simulink subsystem "Attitude_Determination"  (R2022b)
settings: Solver=VariableStepAuto  StartTime=0.0  StopTime=10.0  RelTol=1e-3
undefined symbols (not defined in the file or in its folder): catalogue, sensors, settings
libraries: simulink x1, simulink_extras x1
settings Model: Creator=Nicolò  LastModifiedBy=brent

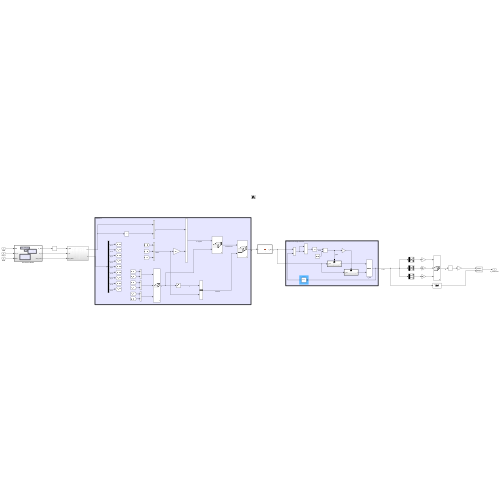
[thumbnail: Simulink's stored preview of the top-level diagram]
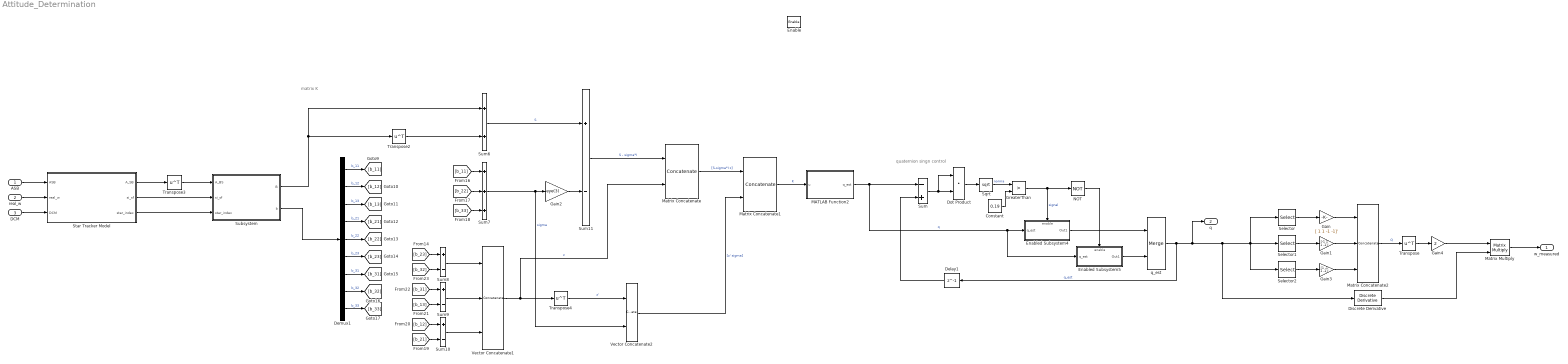
== system Attitude_Determination ==
  note: matrix K
  note: quaternion singn control
  ASB : Inport
  real_w : Inport  Port=2
  DCM : Inport  Port=3
  Enable : EnablePort
  Constant : Constant  Value=0.19
  Delay1 : Delay  DelayLength=1  InitialCondition=settings.q0
  Demux1 : Demux  Outputs=9
  Discrete Derivative : simulink/Discrete/Discrete Derivative  gainval=1.0  ICPrevScaledInput=0  OutMin=[]  OutMax=[]  OutDataType=fixdt(1, 16)  OutScaling=2^-10  DoSatur=off
  Dot Product : DotProduct  OutDataTypeStr=Inherit: Inherit via internal rule
  Enabled Subsystem4 : Subsystem  TreatAsAtomicUnit=on
  Enabled Subsystem5 : Subsystem  TreatAsAtomicUnit=on
  Gain : Gain  Gain=[ 1 1 -1 -1]'
  Gain1 : Gain  Gain=[-1 1 1 -1]'
  Gain2 : Gain  Gain=eye(3)
  Gain3 : Gain  Gain=[1 -1 1 -1]'
  Gain4 : Gain  Gain=2
  GreaterThan : RelationalOperator  Operator=>  OutDataTypeStr=boolean  RndMeth=Simplest  InputSameDT=off
  MATLAB Function2 : MATLAB Function  TreatAsAtomicUnit=on
  Matrix Concatenate : Concatenate  Mode=Multidimensional array  ConcatenateDimension=2
  Matrix Concatenate1 : Concatenate  Mode=Multidimensional array
  Matrix Concatenate2 : Concatenate  NumInputs=3  Mode=Multidimensional array  ConcatenateDimension=2
  Matrix Multiply : Product  Multiplication=Matrix(*)
  NOT : Logic  Operator=NOT  IconShape=distinctive  AllPortsSameDT=off  OutDataTypeStr=boolean
  Selector : Selector  InputPortWidth=4  IndexOptions=Index vector (dialog)  Indices=[4 3 2 1]  OutputSizes=1
  Selector1 : Selector  InputPortWidth=4  IndexOptions=Index vector (dialog)  Indices=[3 4 1 2]  OutputSizes=1
  Selector2 : Selector  InputPortWidth=4  IndexOptions=Index vector (dialog)  Indices=[2 1 4 3]  OutputSizes=1
  Sqrt : Sqrt
  Star Tracker Model : Subsystem  TreatAsAtomicUnit=on
  Subsystem : Subsystem
  Sum : Sum  Inputs=-+
  Sum{8..11} (4 alike) : Sum  Inputs=+-
  Sum6 : Sum
  Sum7 : Sum  Inputs=+++
  Transpose{,2..4} (4 alike) : Math  Operator=transpose
  Vector Concatenate1 : Concatenate  NumInputs=3  Mode=Multidimensional array
  Vector Concatenate2 : Concatenate
  q_est : Merge
  w_measured : Outport
  q : Outport  Port=2
  wires:
  Subsystem/2(b) -> Demux1/1
  Star Tracker Model/3(star_index) -> Subsystem/3(star_index)
  Constant/1 -> GreaterThan/2
  Enabled Subsystem4/1(Out1) -> q_est/1
  Demux1/2 -> [b_12]  "b_12"
  GreaterThan/1 -> NOT/1, Enabled Subsystem4/Enable  "signal"
  Gain2/1 -> Sum11/2
  Matrix Concatenate/1 -> Matrix Concatenate1/1  "[S-sigma*I z]"
  MATLAB Function2/1(q_est) -> Enabled Subsystem4/1(q_est), Enabled Subsystem5/1(q_est), Sum/1  "q"
  Sqrt/1 -> GreaterThan/1  "norma"
  Sum9/1 -> Vector Concatenate1/2
  Dot Product/1 -> Sqrt/1
  [b_32] -> Sum8/2
  Transpose4/1 -> Vector Concatenate2/1  "z'"
  NOT/1 -> Enabled Subsystem5/Enable
  Transpose2/1 -> Sum6/2
  Demux1/7 -> [b_31]  "b_31"
  Demux1/4 -> [b_21]  "b_21"
  Star Tracker Model/1(A_SB) -> Transpose3/1
  Demux1/1 -> [b_11]  "b_11"
  Sum8/1 -> Vector Concatenate1/1
  Transpose3/1 -> Subsystem/1(A_BS)
  [b_23] -> Sum8/1
  Matrix Concatenate1/1 -> MATLAB Function2/1(u)  "K"
  [b_21] -> Sum10/2
  Vector Concatenate1/1 -> Matrix Concatenate/2, Transpose4/1  "z"
  Delay1/1 -> Sum/2
  Demux1/3 -> [b_13]  "b_13"
  [b_13] -> Sum9/2
  Vector Concatenate2/1 -> Matrix Concatenate1/2  "[z' sigma]"
  [b_33] -> Sum7/3
  Sum11/1 -> Matrix Concatenate/1  "S - sigma*I"
  [b_12] -> Sum10/1
  Demux1/8 -> [b_32]  "b_32"
  Sum7/1 -> Vector Concatenate2/2, Gain2/1  "sigma"
  Demux1/9 -> [b_33]  "b_33"
  Demux1/6 -> [b_23]  "b_23"
  Demux1/5 -> [b_22]  "b_22"
  Star Tracker Model/2(si_sf) -> Subsystem/2(si_sf)
  [b_11] -> Sum7/1
  [b_22] -> Sum7/2
  Sum10/1 -> Vector Concatenate1/3
  Sum6/1 -> Sum11/1  "S"
  Subsystem/1(B) -> Sum6/1, Transpose2/1
  Sum/1 -> Dot Product/1, Dot Product/2
  Enabled Subsystem5/1(Out1) -> q_est/2
  [b_31] -> Sum9/1
  Selector2/1 -> Gain3/1
  Discrete Derivative/1 -> Matrix Multiply/2
  q_est/1 -> Discrete Derivative/1, Selector/1, Selector2/1, Selector1/1, q/1, Delay1/1  "q_est"
  Gain3/1 -> Matrix Concatenate2/3
  Matrix Concatenate2/1 -> Transpose/1  "Q"
  Selector/1 -> Gain/1
  Gain4/1 -> Matrix Multiply/1
  Matrix Multiply/1 -> w_measured/1
  Gain/1 -> Matrix Concatenate2/1
  Gain1/1 -> Matrix Concatenate2/2
  Selector1/1 -> Gain1/1
  Transpose/1 -> Gain4/1
  ASB/1 -> Star Tracker Model/1(ASB)
  real_w/1 -> Star Tracker Model/2(real_w)
  DCM/1 -> Star Tracker Model/3(DCM)

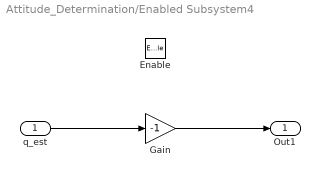
== system Attitude_Determination/Enabled Subsystem4 ==
  q_est : Inport
  Enable : EnablePort
  Gain : Gain  Gain=-1
  Out1 : Outport
  wires:
  q_est/1 -> Gain/1
  Gain/1 -> Out1/1

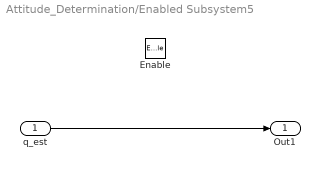
== system Attitude_Determination/Enabled Subsystem5 ==
  q_est : Inport
  Enable : EnablePort
  Out1 : Outport
  wires:
  q_est/1 -> Out1/1

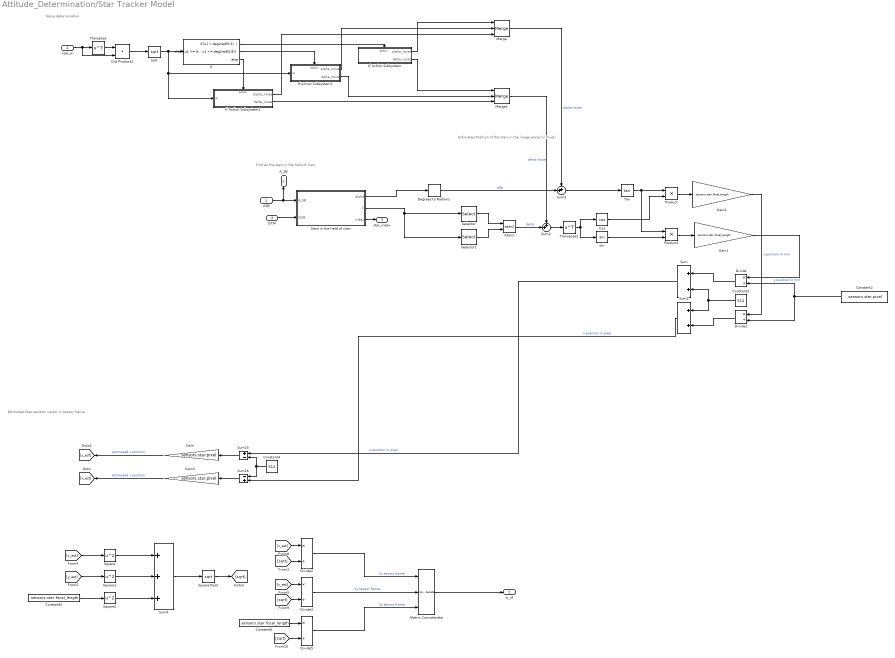
== system Attitude_Determination/Star Tracker Model ==
  note: Estimated Star position vector in Sensor frame
  note: Find all the stars in the field of view
  note: Estimated Position of the stars in the image plane (in Pixel)
  note: Noise determination
  ASB : Inport
  real_w : Inport  Port=2
  DCM : Inport  Port=3
  Atan2 : Trigonometry  Operator=atan2
  Constant2 : Constant  Value=sensors.star.pixel
  Constant3 : Constant  Value=512
  Constant4 : Constant  Value=512
  Constant5 : Constant  Value=sensors.star.focal_length
  Constant6 : Constant  Value=sensors.star.focal_length
  Cos : Trigonometry  Operator=cos
  Degrees to Radians : simulink_extras/Transformations/Degrees to Radians
  Divide{,1..3,5} (5 alike) : Product  Inputs=*/
  Dot Product2 : DotProduct  OutDataTypeStr=Inherit: Inherit via internal rule
  Gain : Gain  Gain=sensors.star.pixel
  Gain1 : Gain  Gain=sensors.star.focal_length
  Gain2 : Gain  Gain=sensors.star.focal_length
  Gain3 : Gain  Gain=sensors.star.pixel
  If : If  IfExpression=u1 < deg2rad(0.3)  ElseIfExpressions="u1 >= deg2rad(0.3) &  u1 <= deg2rad(0.8)"
  If Action Subsystem : Subsystem  TreatAsAtomicUnit=on
  If Action Subsystem1 : Subsystem  TreatAsAtomicUnit=on
  If Action Subsystem2 : Subsystem  TreatAsAtomicUnit=on
  Matrix Concatenate : Concatenate  NumInputs=3  Mode=Multidimensional array  ConcatenateDimension=2
  Merge : Merge  Inputs=3
  Merge1 : Merge  Inputs=3
  Product : Product
  Product1 : Product
  Selector : Selector  NumberOfDimensions=2  InputPortWidth=3  IndexOptions=Index vector (dialog),Index vector (dialog)  Indices=2,[1:10]  OutputSizes=1,1
  Selector1 : Selector  NumberOfDimensions=2  InputPortWidth=3  IndexOptions=Index vector (dialog),Index vector (dialog)  Indices=1,[1:10]  OutputSizes=1,1
  Sin : Trigonometry
  Sqrt : Sqrt
  Square : Math  Operator=square
  Square Root : Sqrt
  Square1 : Math  Operator=square
  Square2 : Math  Operator=square
  Stars in the field of view : MATLAB Function  TreatAsAtomicUnit=on
  Sum : Sum
  Sum1 : Sum
  Sum15 : Sum  Inputs=+-
  Sum16 : Sum  Inputs=-+
  Sum2 : Sum  Inputs=++|
  Sum3 : Sum  Inputs=++|
  Sum4 : Sum  Inputs=+++
  Tan : Trigonometry  Operator=tan
  Transpose : Math  Operator=transpose
  Transpose2 : Math  Operator=transpose
  A_SB : Outport
  si_sf : Outport  Port=2
  star_index : Outport  Port=3
  wires:
  [sqrt] -> Divide2/2
  Dot Product2/1 -> Sqrt/1
  Divide1/1 -> Sum1/2
  Sin/1 -> Product1/2
  If/3 -> If Action Subsystem2/Action
  Stars in the field of view/3(index) -> star_index/1
  [sqrt] -> Divide5/2
  Gain/1 -> [y_est]  "estimated y position"
  Constant6/1 -> Divide5/1
  [sqrt] -> Divide3/2
  Transpose/1 -> Dot Product2/1
  If/1 -> If Action Subsystem/Action
  Gain2/1 -> Divide1/1  "x position in mm"
  real_w/1 -> Transpose/1, Dot Product2/2
  Stars in the field of view/2(S) -> Selector/1, Selector1/1
  Matrix Concatenate/1 -> si_sf/1
  Square Root/1 -> [sqrt]
  Selector/1 -> Atan2/1
  Transpose2/1 -> Cos/1, Sin/1
  Divide5/1 -> Matrix Concatenate/3  "Sz sensor frame"
  Selector1/1 -> Atan2/2
  Divide2/1 -> Matrix Concatenate/1  "Sx sensor frame"
  Sum4/1 -> Square Root/1
  Sum/1 -> Sum15/1  "y position in pixel"
  Square2/1 -> Sum4/3
  Sum15/1 -> Gain/1
  [y_est] -> Square1/1
  Square/1 -> Sum4/1
  [x_est] -> Divide2/1
  Gain3/1 -> [x_est]  "estimated x position"
  Sum16/1 -> Gain3/1
  Constant3/1 -> Sum1/1, Sum/2
  Sum3/1 -> Tan/1
  Sum2/1 -> Transpose2/1
  Square1/1 -> Sum4/2
  Sum1/1 -> Sum16/2  "x position in pixel"
  Constant5/1 -> Square2/1
  If/2 -> If Action Subsystem1/Action
  Gain1/1 -> Divide/1  "y position in mm"
  Tan/1 -> Product/1, Product1/1
  Atan2/1 -> Sum2/2  "delta"
  [x_est] -> Square/1
  DCM/1 -> Stars in the field of view/2(DCM)
  Stars in the field of view/1(alpha) -> Degrees to Radians/1
  Product1/1 -> Gain1/1
  Degrees to Radians/1 -> Sum3/2  "alfa"
  Constant2/1 -> Divide1/2, Divide/2
  Product/1 -> Gain2/1
  Divide3/1 -> Matrix Concatenate/2  "Sy sensor frame"
  Divide/1 -> Sum/1
  Constant4/1 -> Sum16/1, Sum15/2
  Sqrt/1 -> If Action Subsystem2/1(w), If Action Subsystem1/1(w), If/1
  Cos/1 -> Product/2
  [y_est] -> Divide3/1
  ASB/1 -> Stars in the field of view/1(A_SB), A_SB/1
  If Action Subsystem2/1(alpha_noise) -> Merge/3
  If Action Subsystem1/1(alpha_noise) -> Merge/2
  If Action Subsystem/1(alpha_noise) -> Merge/1
  If Action Subsystem/2(delta_noise) -> Merge1/1
  If Action Subsystem1/2(delta_noise) -> Merge1/2
  If Action Subsystem2/2(delta_noise) -> Merge1/3
  Merge/1 -> Sum3/1  "alpha noise"
  Merge1/1 -> Sum2/1  "delta noise"

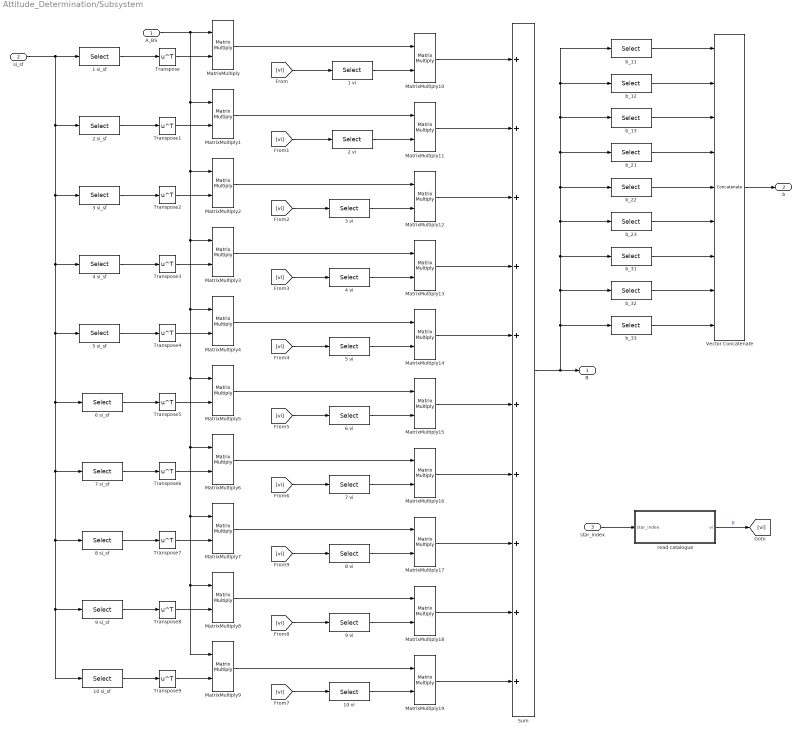
== system Attitude_Determination/Subsystem ==
  A_BS : Inport
  si_sf : Inport  Port=2
  star_index : Inport  Port=3
  1 si_sf : Selector  NumberOfDimensions=2  InputPortWidth=3  IndexOptions=Index vector (dialog),Select all  Indices=1,1  OutputSizes=1,1
  1 vi : Selector  NumberOfDimensions=2  InputPortWidth=3  IndexOptions=Index vector (dialog),Select all  Indices=1,1  OutputSizes=1,1
  10 si_sf : Selector  NumberOfDimensions=2  InputPortWidth=3  IndexOptions=Index vector (dialog),Select all  Indices=10,1  OutputSizes=1,1
  10 vi : Selector  NumberOfDimensions=2  InputPortWidth=3  IndexOptions=Index vector (dialog),Select all  Indices=10,1  OutputSizes=1,1
  2 si_sf : Selector  NumberOfDimensions=2  InputPortWidth=3  IndexOptions=Index vector (dialog),Select all  Indices=2,1  OutputSizes=1,1
  2 vi : Selector  NumberOfDimensions=2  InputPortWidth=3  IndexOptions=Index vector (dialog),Select all  Indices=2,1  OutputSizes=1,1
  3 si_sf : Selector  NumberOfDimensions=2  InputPortWidth=3  IndexOptions=Index vector (dialog),Select all  Indices=3,1  OutputSizes=1,1
  3 vi : Selector  NumberOfDimensions=2  InputPortWidth=3  IndexOptions=Index vector (dialog),Select all  Indices=3,1  OutputSizes=1,1
  4 si_sf : Selector  NumberOfDimensions=2  InputPortWidth=3  IndexOptions=Index vector (dialog),Select all  Indices=4,1  OutputSizes=1,1
  4 vi : Selector  NumberOfDimensions=2  InputPortWidth=3  IndexOptions=Index vector (dialog),Select all  Indices=4,1  OutputSizes=1,1
  5 si_sf : Selector  NumberOfDimensions=2  InputPortWidth=3  IndexOptions=Index vector (dialog),Select all  Indices=5,1  OutputSizes=1,1
  5 vi : Selector  NumberOfDimensions=2  InputPortWidth=3  IndexOptions=Index vector (dialog),Select all  Indices=5,1  OutputSizes=1,1
  6 si_sf : Selector  NumberOfDimensions=2  InputPortWidth=3  IndexOptions=Index vector (dialog),Select all  Indices=6,1  OutputSizes=1,1
  6 vi : Selector  NumberOfDimensions=2  InputPortWidth=3  IndexOptions=Index vector (dialog),Select all  Indices=6,1  OutputSizes=1,1
  7 si_sf : Selector  NumberOfDimensions=2  InputPortWidth=3  IndexOptions=Index vector (dialog),Select all  Indices=7,1  OutputSizes=1,1
  7 vi : Selector  NumberOfDimensions=2  InputPortWidth=3  IndexOptions=Index vector (dialog),Select all  Indices=7,1  OutputSizes=1,1
  8 si_sf : Selector  NumberOfDimensions=2  InputPortWidth=3  IndexOptions=Index vector (dialog),Select all  Indices=8,1  OutputSizes=1,1
  8 vi : Selector  NumberOfDimensions=2  InputPortWidth=3  IndexOptions=Index vector (dialog),Select all  Indices=8,1  OutputSizes=1,1
  9 si_sf : Selector  NumberOfDimensions=2  InputPortWidth=3  IndexOptions=Index vector (dialog),Select all  Indices=9,1  OutputSizes=1,1
  9 vi : Selector  NumberOfDimensions=2  InputPortWidth=3  IndexOptions=Index vector (dialog),Select all  Indices=9,1  OutputSizes=1,1
  MatrixMultiply{,1..19} (20 alike) : Product  Multiplication=Matrix(*)
  Sum : Sum  Inputs=++++++++++
  Transpose{,1..9} (10 alike) : Math  Operator=transpose
  Vector Concatenate : Concatenate  NumInputs=9
  b_11 : Selector  NumberOfDimensions=2  InputPortWidth=3  IndexOptions=Index vector (dialog),Index vector (dialog)  Indices=1,1  OutputSizes=1,1
  b_12 : Selector  NumberOfDimensions=2  InputPortWidth=3  IndexOptions=Index vector (dialog),Index vector (dialog)  Indices=1,2  OutputSizes=1,1
  b_13 : Selector  NumberOfDimensions=2  InputPortWidth=3  IndexOptions=Index vector (dialog),Index vector (dialog)  Indices=1,3  OutputSizes=1,1
  b_21 : Selector  NumberOfDimensions=2  InputPortWidth=3  IndexOptions=Index vector (dialog),Index vector (dialog)  Indices=2,1  OutputSizes=1,1
  b_22 : Selector  NumberOfDimensions=2  InputPortWidth=3  IndexOptions=Index vector (dialog),Index vector (dialog)  Indices=2,2  OutputSizes=1,1
  b_23 : Selector  NumberOfDimensions=2  InputPortWidth=3  IndexOptions=Index vector (dialog),Index vector (dialog)  Indices=2,3  OutputSizes=1,1
  b_31 : Selector  NumberOfDimensions=2  InputPortWidth=3  IndexOptions=Index vector (dialog),Index vector (dialog)  Indices=3,1  OutputSizes=1,1
  b_32 : Selector  NumberOfDimensions=2  InputPortWidth=3  IndexOptions=Index vector (dialog),Index vector (dialog)  Indices=3,2  OutputSizes=1,1
  b_33 : Selector  NumberOfDimensions=2  InputPortWidth=3  IndexOptions=Index vector (dialog),Index vector (dialog)  Indices=3,3  OutputSizes=1,1
  read catalogue : MATLAB Function  TreatAsAtomicUnit=on
  B : Outport
  b : Outport  Port=2
  wires:
  A_BS/1 -> MatrixMultiply1/1, MatrixMultiply2/1, MatrixMultiply5/1, MatrixMultiply6/1, MatrixMultiply7/1, MatrixMultiply9/1, MatrixMultiply8/1, MatrixMultiply4/1, MatrixMultiply3/1, MatrixMultiply/1
  star_index/1 -> read catalogue/1(star_index)
  si_sf/1 -> 1 si_sf/1, 3 si_sf/1, 5 si_sf/1, 7 si_sf/1, 8 si_sf/1, 9 si_sf/1, 10 si_sf/1, 6 si_sf/1, 4 si_sf/1, 2 si_sf/1
  1 si_sf/1 -> Transpose/1
  Transpose/1 -> MatrixMultiply/2
  9 si_sf/1 -> Transpose8/1
  10 si_sf/1 -> Transpose9/1
  8 si_sf/1 -> Transpose7/1
  7 si_sf/1 -> Transpose6/1
  6 si_sf/1 -> Transpose5/1
  5 si_sf/1 -> Transpose4/1
  2 si_sf/1 -> Transpose1/1
  3 si_sf/1 -> Transpose2/1
  4 si_sf/1 -> Transpose3/1
  Transpose3/1 -> MatrixMultiply3/2
  Transpose1/1 -> MatrixMultiply1/2
  Transpose2/1 -> MatrixMultiply2/2
  Transpose4/1 -> MatrixMultiply4/2
  Transpose5/1 -> MatrixMultiply5/2
  Transpose6/1 -> MatrixMultiply6/2
  Transpose7/1 -> MatrixMultiply7/2
  Transpose8/1 -> MatrixMultiply8/2
  Transpose9/1 -> MatrixMultiply9/2
  MatrixMultiply1/1 -> MatrixMultiply11/1
  MatrixMultiply2/1 -> MatrixMultiply12/1
  MatrixMultiply/1 -> MatrixMultiply10/1
  MatrixMultiply5/1 -> MatrixMultiply15/1
  MatrixMultiply4/1 -> MatrixMultiply14/1
  MatrixMultiply3/1 -> MatrixMultiply13/1
  MatrixMultiply8/1 -> MatrixMultiply18/1
  MatrixMultiply7/1 -> MatrixMultiply17/1
  MatrixMultiply6/1 -> MatrixMultiply16/1
  MatrixMultiply9/1 -> MatrixMultiply19/1
  read catalogue/1(vi) -> [vi]  "B"
  [vi] -> 3 vi/1
  [vi] -> 2 vi/1
  [vi] -> 4 vi/1
  [vi] -> 5 vi/1
  [vi] -> 6 vi/1
  [vi] -> 7 vi/1
  [vi] -> 10 vi/1
  [vi] -> 9 vi/1
  [vi] -> 8 vi/1
  MatrixMultiply11/1 -> Sum/2
  MatrixMultiply12/1 -> Sum/3
  MatrixMultiply13/1 -> Sum/4
  MatrixMultiply14/1 -> Sum/5
  MatrixMultiply15/1 -> Sum/6
  MatrixMultiply16/1 -> Sum/7
  MatrixMultiply17/1 -> Sum/8
  MatrixMultiply18/1 -> Sum/9
  MatrixMultiply19/1 -> Sum/10
  Sum/1 -> b_33/1, b_32/1, b_31/1, b_23/1, b_12/1, b_11/1, b_13/1, b_21/1, b_22/1, B/1
  MatrixMultiply10/1 -> Sum/1
  [vi] -> 1 vi/1
  b_11/1 -> Vector Concatenate/1
  b_12/1 -> Vector Concatenate/2
  b_13/1 -> Vector Concatenate/3
  b_21/1 -> Vector Concatenate/4
  b_22/1 -> Vector Concatenate/5
  b_23/1 -> Vector Concatenate/6
  b_31/1 -> Vector Concatenate/7
  b_32/1 -> Vector Concatenate/8
  b_33/1 -> Vector Concatenate/9
  Vector Concatenate/1 -> b/1
  1 vi/1 -> MatrixMultiply10/2
  2 vi/1 -> MatrixMultiply11/2
  3 vi/1 -> MatrixMultiply12/2
  4 vi/1 -> MatrixMultiply13/2
  5 vi/1 -> MatrixMultiply14/2
  6 vi/1 -> MatrixMultiply15/2
  7 vi/1 -> MatrixMultiply16/2
  8 vi/1 -> MatrixMultiply17/2
  9 vi/1 -> MatrixMultiply18/2
  10 vi/1 -> MatrixMultiply19/2

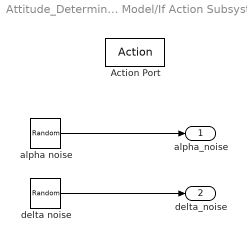
== system Attitude_Determination/Star Tracker Model/If Action Subsystem ==
  Action Port : ActionPort
  "alpha noise " : RandomNumber  Variance=sensors.star.alpha_err  Seed=1687
  delta noise : RandomNumber  Variance=sensors.star.delta_err  Seed=798
  alpha_noise : Outport
  delta_noise : Outport  Port=2
  wires:
  "alpha noise "/1 -> alpha_noise/1
  delta noise/1 -> delta_noise/1

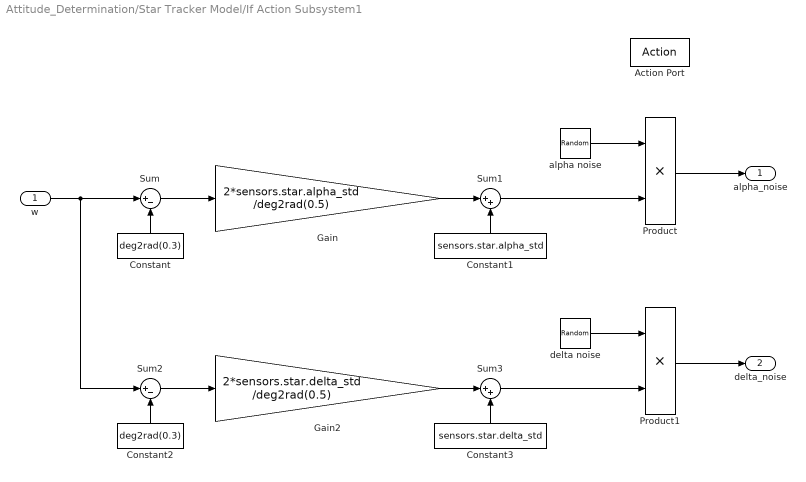
== system Attitude_Determination/Star Tracker Model/If Action Subsystem1 ==
  w : Inport
  Action Port : ActionPort
  Constant : Constant  Value=deg2rad(0.3)
  Constant1 : Constant  Value=sensors.star.alpha_std
  Constant2 : Constant  Value=deg2rad(0.3)
  Constant3 : Constant  Value=sensors.star.delta_std
  Gain : Gain  Gain=2*sensors.star.alpha_std /deg2rad(0.5)
  Gain2 : Gain  Gain=2*sensors.star.delta_std /deg2rad(0.5)
  Product : Product
  Product1 : Product
  Sum : Sum  Inputs=|+-
  Sum1 : Sum  Inputs=|++
  Sum2 : Sum  Inputs=|+-
  Sum3 : Sum  Inputs=|++
  "alpha noise " : RandomNumber  Seed=1687
  delta noise : RandomNumber  Seed=798
  alpha_noise : Outport
  delta_noise : Outport  Port=2
  wires:
  "alpha noise "/1 -> Product/1
  Constant/1 -> Sum/2
  Sum/1 -> Gain/1
  Gain/1 -> Sum1/1
  Constant1/1 -> Sum1/2
  Sum1/1 -> Product/2
  Product/1 -> alpha_noise/1
  Product1/1 -> delta_noise/1
  Sum3/1 -> Product1/2
  Constant3/1 -> Sum3/2
  Gain2/1 -> Sum3/1
  Sum2/1 -> Gain2/1
  Constant2/1 -> Sum2/2
  w/1 -> Sum2/1, Sum/1
  delta noise/1 -> Product1/1

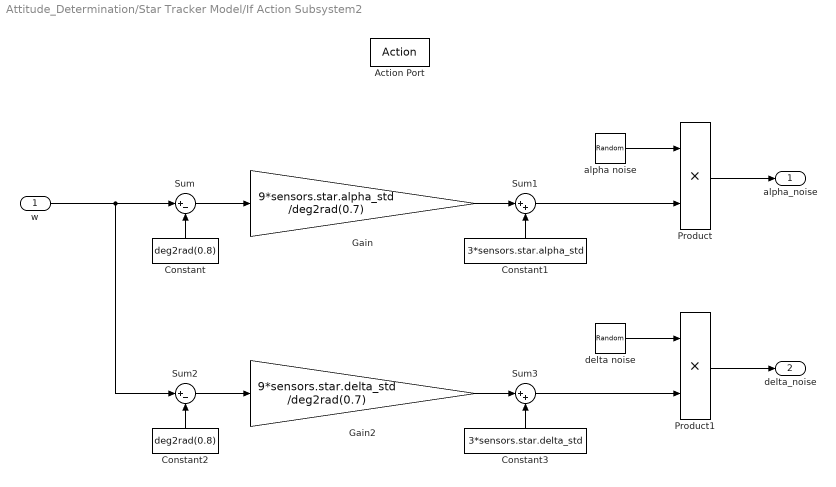
== system Attitude_Determination/Star Tracker Model/If Action Subsystem2 ==
  w : Inport
  Action Port : ActionPort
  Constant : Constant  Value=deg2rad(0.8)
  Constant1 : Constant  Value=3*sensors.star.alpha_std
  Constant2 : Constant  Value=deg2rad(0.8)
  Constant3 : Constant  Value=3*sensors.star.delta_std
  Gain : Gain  Gain=9*sensors.star.alpha_std /deg2rad(0.7)
  Gain2 : Gain  Gain=9*sensors.star.delta_std /deg2rad(0.7)
  Product : Product
  Product1 : Product
  Sum : Sum  Inputs=|+-
  Sum1 : Sum  Inputs=|++
  Sum2 : Sum  Inputs=|+-
  Sum3 : Sum  Inputs=|++
  "alpha noise " : RandomNumber  Seed=1687
  delta noise : RandomNumber  Seed=798
  alpha_noise : Outport
  delta_noise : Outport  Port=2
  wires:
  Sum2/1 -> Gain2/1
  Sum3/1 -> Product1/2
  Sum/1 -> Gain/1
  "alpha noise "/1 -> Product/1
  Constant2/1 -> Sum2/2
  Gain2/1 -> Sum3/1
  Constant1/1 -> Sum1/2
  Sum1/1 -> Product/2
  Gain/1 -> Sum1/1
  Product/1 -> alpha_noise/1
  Constant3/1 -> Sum3/2
  w/1 -> Sum2/1, Sum/1
  Product1/1 -> delta_noise/1
  Constant/1 -> Sum/2
  delta noise/1 -> Product1/1

== matlab function Attitude_Determination/Star Tracker Model/Stars in the field of view ==
  data: alpha output; S output; sensors parameter; catalogue parameter; A_SB input; DCM input; index output
function [alpha,S,index] = findVisibleStars(sensors,catalogue,A_SB,DCM)
%{
    This function takes as an input the star catalogue, the star sensor
    parameters and the current attitude to find the list of visible stars
%}

index = zeros(10,1);

S = sensors.star.S;
alpha = sensors.star.alpha;

i = 1;
j = 1;

while j<=10

    % star's normalized position vector in sensor frame
    S_temp = A_SB*DCM*(catalogue(i,1:3))';
 
    % angle between star's position vector and sensor's pointing axis
    alpha_temp = acos( dot(S_temp,[0;0;1]) );
    alpha_temp = rad2deg(alpha_temp);
    % check if star is in field of view
    if alpha_temp <= sensors.star.fov/2

        S(:,j) = [S_temp;i];
        index (j) = i;
        alpha(j) = alpha_temp;
        j = j + 1;
    end
    i= i+1;
end

== matlab function Attitude_Determination/Subsystem/read catalogue ==
  data: vi output; star_index input; catalogue parameter
function vi  = starCoordinates(star_index, catalogue)

vi = zeros(length(star_index), 3);

% vector of real star position
for k = 1:length(star_index)

    % check if the sensor is pointing correctly
    if star_index(k) == 0
        vi(k, :) = zeros(3,1);
    else
        vi(k, :) = catalogue(star_index(k), (1:3));
        vi(k, :) = vi(k, :)/(norm(vi(k, :)));
    end

end

== matlab function Attitude_Determination/MATLAB Function2 ==
  data: u input; q_est output
function q_est  = fcn(u)

[q, lambda] = eig(u);
lambda_est = [lambda(1,1) lambda(2,2) lambda(3,3) lambda(4,4)];
[m, i] = max(real(lambda_est));
q_est = real(q(:, i));
